simulink model "Wind_Turbine_Modeling_01"  (R2024a)
settings: Solver=VariableStepAuto  StartTime=0.0  StopTime=10.0  RelTol=1e-3
libraries: spspowerguiLib x1
settings Model: Creator=mansur  LastModifiedBy=mansur

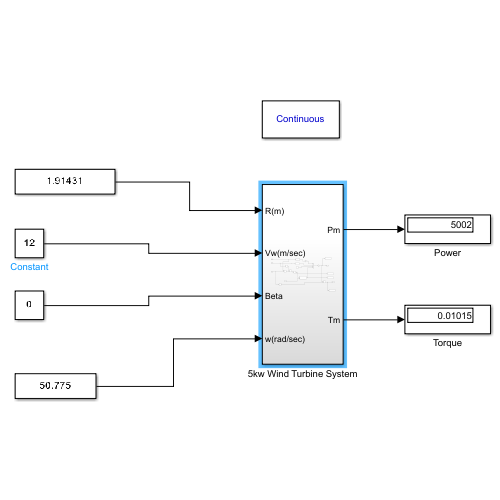
[thumbnail: Simulink's stored preview of the top-level diagram]
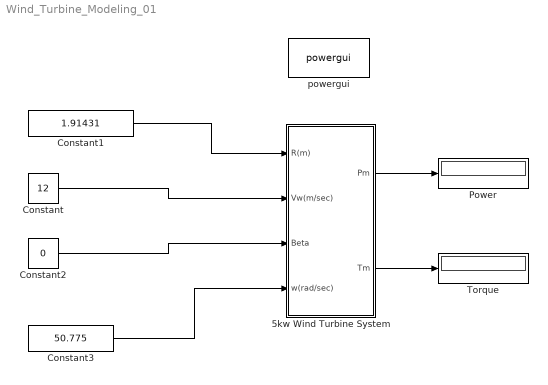
== system Wind_Turbine_Modeling_01 ==
  5kw Wind Turbine System : Subsystem
  Constant : Constant  Value=12
  Constant1 : Constant  Value=1.91431
  Constant2 : Constant  Value=0
  Constant3 : Constant  Value=50.775
  Power : Display
  Torque : Display
  powergui : spspowerguiLib/powergui  Priority=1  SimulationMode=Continuous  SampleTime=50e-6  frequency=60  Iterations=50  frequencyindice=60  Pbase=100e6  ErrMax=1e-4  UnitsV=kV  UnitsW=MW  buscounter=0  FunctionMessages=off  echomessages=off  EnableUseOfTLC=off  CurrentSourceSwitches=off  DisableSnubberDevices=off  DisableRonSwitches=off  DisableVfSwitches=off  DisplayEquations=off  AutomaticDiscreteSolvers=off  SolverType=Tustin/Backward Euler (TBE)  Interpol=off  ExternalGateDelay=off  methode=off  Ts=100  x0status=blocks  SPID=on  SwTol=0  HookPort=off  NonlinearTolerance=1e-4  nMaxIteration=100  ContinueOnMaxIteration=off  RestoreLinks=warning  ResistiveCurrentMeasurement=off  Frange=[0:2:500]  Ylog=off  Xlog=on  ShowGrid=off  save=off  variable=ZData  structure=0  ZoomFFT=off  StartTime=0.0  cycles=1  DisplayStyle=1  fundamental=60  FreqAxis=off  MaxFrequency=1000  frequencyindicesteady=1  RmsSteady=1  display=off
  wires:
  Constant1/1 -> 5kw Wind Turbine System/1(R(m))
  Constant/1 -> 5kw Wind Turbine System/2(Vw(m/sec))
  Constant2/1 -> 5kw Wind Turbine System/3(Beta)
  Constant3/1 -> 5kw Wind Turbine System/4(w(rad/sec))
  5kw Wind Turbine System/2(Tm) -> Torque/1
  5kw Wind Turbine System/1(Pm) -> Power/1

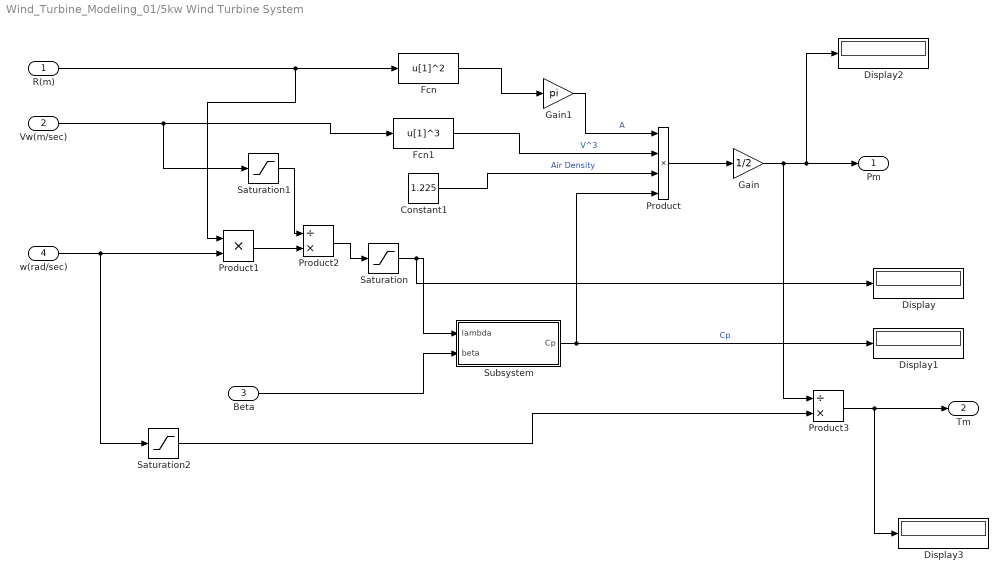
== system Wind_Turbine_Modeling_01/5kw Wind Turbine System ==
  R(m) : Inport
  Vw(m/sec) : Inport  Port=2
  Beta : Inport  Port=3
  w(rad/sec) : Inport  Port=4
  Constant1 : Constant  Value=1.225
  Display{,1..3} (4 alike) : Display
  Fcn : Fcn  Expr=u[1]^2
  Fcn1 : Fcn  Expr=u[1]^3
  Gain : Gain  Gain=1/2
  Gain1 : Gain  Gain=pi
  Product : Product  Inputs=4
  Product1 : Product
  Product2 : Product  Inputs=/*
  Product3 : Product  Inputs=/*
  Saturation : Saturate  UpperLimit=inf  LowerLimit=1e-6
  Saturation1 : Saturate  UpperLimit=inf  LowerLimit=1e-6
  Saturation2 : Saturate  UpperLimit=inf  LowerLimit=1e-6
  Subsystem : Subsystem
  Pm : Outport
  Tm : Outport  Port=2
  wires:
  Gain/1 -> Product3/1, Display2/1, Pm/1
  Product/1 -> Gain/1
  Gain1/1 -> Product/1  "A"
  Fcn1/1 -> Product/2  "V^3"
  Constant1/1 -> Product/3  "Air Density"
  Subsystem/1(Cp) -> Product/4, Display1/1  "Cp"
  Fcn/1 -> Gain1/1
  R(m)/1 -> Product1/1, Fcn/1
  Vw(m/sec)/1 -> Saturation1/1, Fcn1/1
  Beta/1 -> Subsystem/2(beta)
  w(rad/sec)/1 -> Saturation2/1, Product1/2
  Product1/1 -> Product2/2
  Product2/1 -> Saturation/1
  Saturation/1 -> Display/1, Subsystem/1(lambda)
  Saturation1/1 -> Product2/1
  Saturation2/1 -> Product3/2
  Product3/1 -> Display3/1, Tm/1

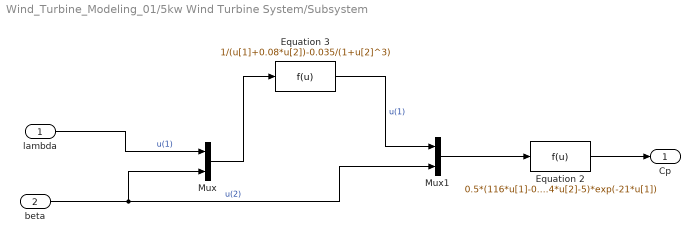
== system Wind_Turbine_Modeling_01/5kw Wind Turbine System/Subsystem ==
  lambda : Inport
  beta : Inport  Port=2
  Equation 2 : Fcn  Expr=0.5*(116*u[1]-0.4*u[2]-5)*exp(-21*u[1])
  Equation 3 : Fcn  Expr=1/(u[1]+0.08*u[2])-0.035/(1+u[2]^3)
  Mux : Mux  Inputs=2
  Mux1 : Mux  Inputs=2
  Cp : Outport
  wires:
  lambda/1 -> Mux/1  "u(1)"
  Equation 2/1 -> Cp/1
  Mux1/1 -> Equation 2/1
  Equation 3/1 -> Mux1/1  "u(1)"
  beta/1 -> Mux1/2, Mux/2  "u(2)"
  Mux/1 -> Equation 3/1
